simulink model "chap1_3n"  (Simulink 6.3)
settings: Solver=ode45  StartTime=0.0  StopTime=10.0  RelTol=1e-3
libraries: simulink x1
settings Model: LastModifiedBy=Administrator  ExtModeTrigMode=oneshot  ExtModeArmWhenConnect=off  StrictBusMsg=None
settings DataIOCC: LimitDataPoints=off  SignalLoggingName=sigsOut
settings OptimizationCC: BooleanDataType=off
settings DebuggingCC: SolverPrmCheckMsg=none
settings HardwareCC: TargetUnknown=on

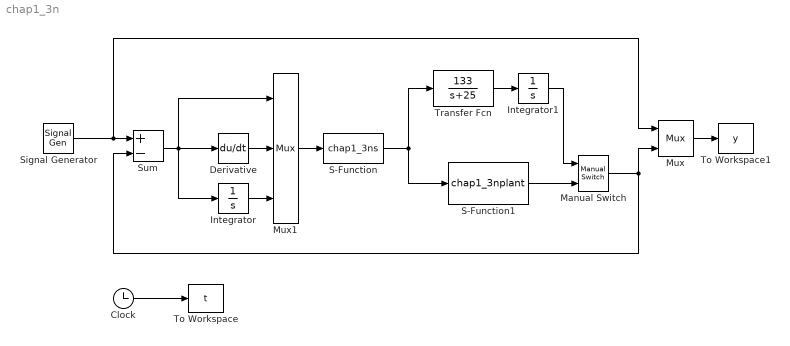
== system chap1_3n ==
  Clock : Clock
      settings: Decimation=10
  Derivative : Derivative
  Integrator : Integrator
  Integrator1 : Integrator
  Manual Switch : simulink/Signal Routing/Manual Switch  sw=0  action=0
  Mux : Mux  Inputs=2
  Mux1 : Mux  Inputs=3
  S-Function : S-Function  FunctionName=chap1_3ns
  S-Function1 : S-Function  FunctionName=chap1_3nplant
  Signal Generator : SignalGenerator  Frequency=0.2
  Sum : Sum  Inputs=+-  SaturateOnIntegerOverflow=on  InputSameDT=on
  To Workspace : ToWorkspace  VariableName=t  SampleTime=-1  SaveFormat=Array
  To Workspace1 : ToWorkspace  VariableName=y  SampleTime=-1  SaveFormat=Array
  Transfer Fcn : TransferFcn  Numerator=[133]  Denominator=[1 25]
  wires:
  Signal Generator/1 -> Sum/1, Mux/1
  Mux/1 -> To Workspace1/1
  Manual Switch/1 -> Mux/2, Sum/2
  Mux1/1 -> S-Function/1
  Derivative/1 -> Mux1/2
  Integrator/1 -> Mux1/3
  Sum/1 -> Mux1/1, Derivative/1, Integrator/1
  Transfer Fcn/1 -> Integrator1/1
  Integrator1/1 -> Manual Switch/1
  S-Function1/1 -> Manual Switch/2
  S-Function/1 -> Transfer Fcn/1, S-Function1/1
  Clock/1 -> To Workspace/1
